simulink model "Distribution_Library"  (Simulink 8.3)
settings: Solver=VariableStepDiscrete  StartTime=0.0  StopTime=100.0  RelTol=1e-3
libraries: simeventslib x4
settings Model: Creator=tsprock3  LastModifiedBy=tsprock3  CovSFcnEnable=on
settings OptimizationCC: ExpressionDepthLimit=2147483647
settings DebuggingCC: FcnCallInpInsideContextMsg=EnableAllAsWarning  FrameProcessingCompatibilityMsg=error  SimStateOlderReleaseMsg=warning
settings GRTTargetCC: CombineOutputUpdateFcns=on  GRTInterface=off

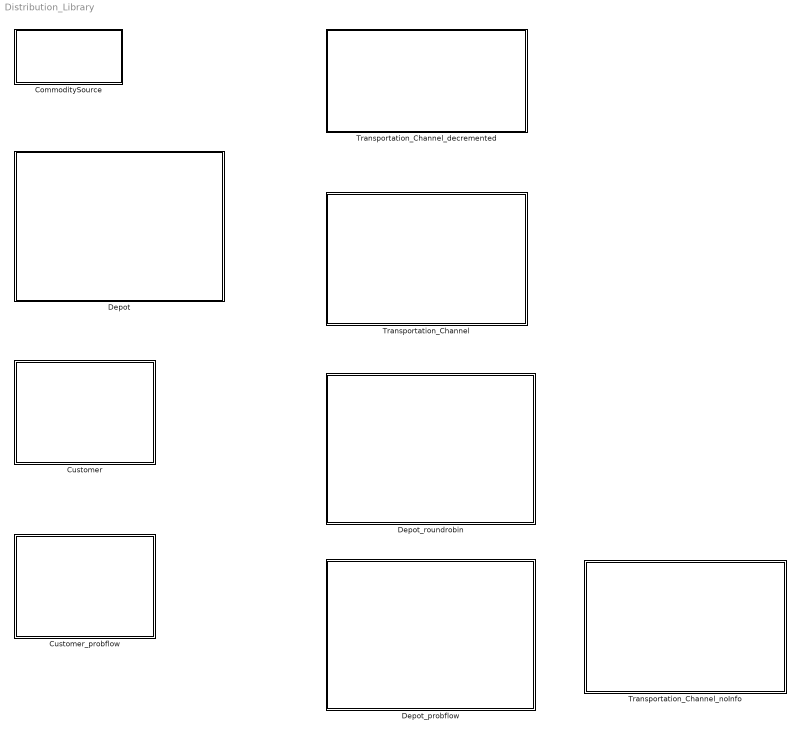
== system Distribution_Library ==
  CommoditySource : Subsystem  mask{Mean=1000/913, AttributeValue=[1 10 9 2]|1|2|1}
      mask prompts: Mean "Frequency"; AttributeValue "Attributes"
      mask TypeOptions Mean: Source/Mean
      mask TypeOptions AttributeValue: setAttribute/AttributeValue
  Customer : Subsystem
  Customer_probflow : Subsystem
  Depot : Subsystem
  Depot_probflow : Subsystem
  Depot_roundrobin : Subsystem
  Transportation_Channel : Subsystem
  Transportation_Channel_decremented : Subsystem
  Transportation_Channel_noInfo : Subsystem

== system Distribution_Library/CommoditySource ==
  Clock : Clock
  Source : TimeBasedEntityGenerator  Distribution=Exponential  InitialSeed=18340  Mean=Mean  GenerateEntityAtSimulationStart=off
  Timed to Event Signal : TimedToEventSignal
  setAttribute : SetAttribute  AttributeName=Route|Origin|Destination|Start  AttributeFrom=Dialog|Dialog|Dialog|Signal port  AttributeValue=[1 10 9 2]|1|2|1  AttributeTreatAsVector=0|1|1|1  EvaluatedAttributeValue={[1 10 9 2];1;2;[]}
      settings: InputPortMap=u3
  OUT_Commodity : PMIOPort  Port=1  Side=Right
  wires:
  Clock/1 -> Timed to Event Signal/1
  Timed to Event Signal/1 -> setAttribute/1
  connections:
  Source/RConn1 -- setAttribute/LConn1
  OUT_Commodity/RConn1 -- setAttribute/RConn1

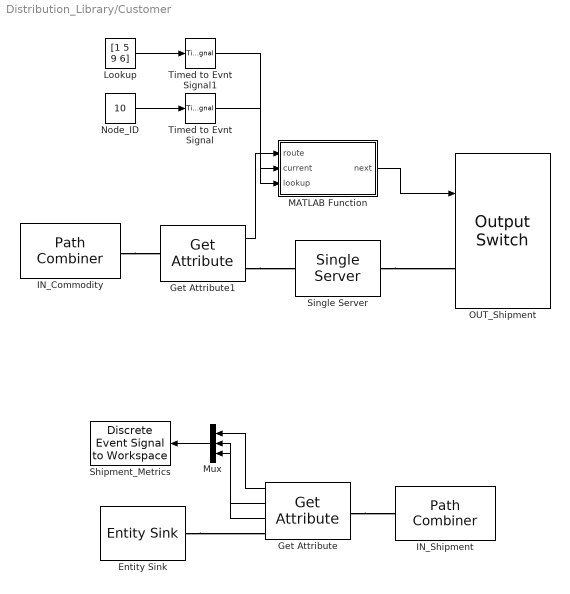
== system Distribution_Library/Customer ==
  Entity Sink : EntitySink
  Get Attribute : GetAttribute  AttributeName=Origin|Destination|Start  AttributeMissing=Error|Error|Error  AttributeDefaultValue=1|1|1  AttributeTreatAsVector=1|1|1  AttributeSendTiming=After entity departure|After entity departure|After entity departure  EvaluatedDefaultAttributeValue={[];[];[]}
      settings: OutputPortMap=o1,o2,o3
  Get Attribute1 : GetAttribute  AttributeName=Route  EvaluatedDefaultAttributeValue={[]}
      settings: OutputPortMap=o1
  IN_Commodity : PathCombiner  NumberInputPorts=4
  IN_Shipment : PathCombiner  NumberInputPorts=1
  Lookup : Constant  Value=[1 5 9 6]
  MATLAB Function : MATLAB Function  TreatAsAtomicUnit=on
  Mux : Mux  Inputs=3
  Node_ID : Constant  Value=10
  OUT_Shipment : OutputSwitch  NumberOutputPorts=1  SwitchingCriterion=From signal port p  AttributeName=Customer
  Shipment_Metrics : simeventslib/SimEvents Sinks/Discrete Event Signal to Workspace  VariableName=Customer_1  SaveFormat=Structure With Time  isMonitorOnly=off  isRecordIC=off
  Single Server : SingleServer  ServiceTime=0
  Timed to Evnt Signal : TimedToEventSignal
  Timed to Evnt Signal1 : TimedToEventSignal
  wires:
  Get Attribute/1 -> Mux/1
  Get Attribute/2 -> Mux/2
  Get Attribute/3 -> Mux/3
  Mux/1 -> Shipment_Metrics/1
  Node_ID/1 -> Timed to Evnt Signal/1
  MATLAB Function/1(next) -> OUT_Shipment/1
  Get Attribute1/1 -> MATLAB Function/1(route)
  Timed to Evnt Signal/1 -> MATLAB Function/2(current)
  Lookup/1 -> Timed to Evnt Signal1/1
  Timed to Evnt Signal1/1 -> MATLAB Function/3(lookup)
  connections:
  Entity Sink/LConn1 -- Get Attribute/RConn1
  Get Attribute/LConn1 -- IN_Shipment/RConn1
  IN_Commodity/RConn1 -- Get Attribute1/LConn1
  Get Attribute1/RConn1 -- Single Server/LConn1
  Single Server/RConn1 -- OUT_Shipment/LConn1

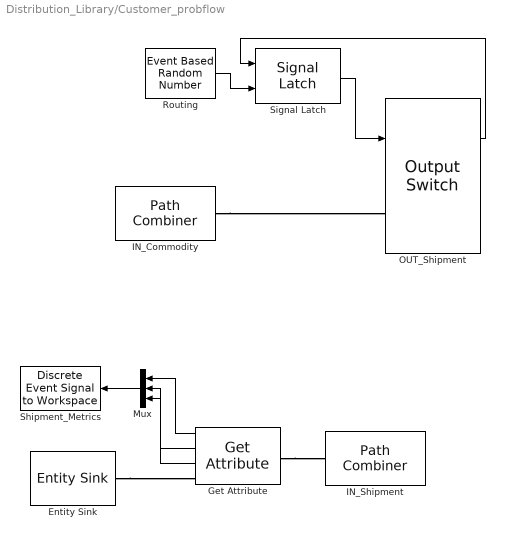
== system Distribution_Library/Customer_probflow ==
  Entity Sink : EntitySink
  Get Attribute : GetAttribute  AttributeName=Origin|Destination|Start  AttributeMissing=Error|Error|Error  AttributeDefaultValue=1|1|1  AttributeTreatAsVector=1|1|1  AttributeSendTiming=After entity departure|After entity departure|After entity departure  EvaluatedDefaultAttributeValue={[];[];[]}
      settings: OutputPortMap=o1,o2,o3
  IN_Commodity : PathCombiner  NumberInputPorts=1
  IN_Shipment : PathCombiner  NumberInputPorts=1
  Mux : Mux  Inputs=3
  OUT_Shipment : OutputSwitch  NumberOutputPorts=1  SwitchingCriterion=From signal port p  AttributeName=Customer  StatNumberDeparted=on
  Routing : EventBasedRandomNumber  Distribution=Arbitrary discrete  valueVecDisc=[1 2]  probVecDisc=[0.1892 0.8108]
  Shipment_Metrics : simeventslib/SimEvents Sinks/Discrete Event Signal to Workspace  VariableName=Customer_1  SaveFormat=Structure With Time  isMonitorOnly=off  isRecordIC=off
  Signal Latch : SignalLatch  InitialMemoryValue=1  ReadMemoryUpon=Write to memory event
      settings: InputPortMap=u0,u2  OutputPortMap=o2
  wires:
  Get Attribute/1 -> Mux/1
  Get Attribute/2 -> Mux/2
  Get Attribute/3 -> Mux/3
  Mux/1 -> Shipment_Metrics/1
  Routing/1 -> Signal Latch/2
  OUT_Shipment/1 -> Signal Latch/1
  Signal Latch/1 -> OUT_Shipment/1
  connections:
  Entity Sink/LConn1 -- Get Attribute/RConn1
  Get Attribute/LConn1 -- IN_Shipment/RConn1
  IN_Commodity/RConn1 -- OUT_Shipment/LConn1

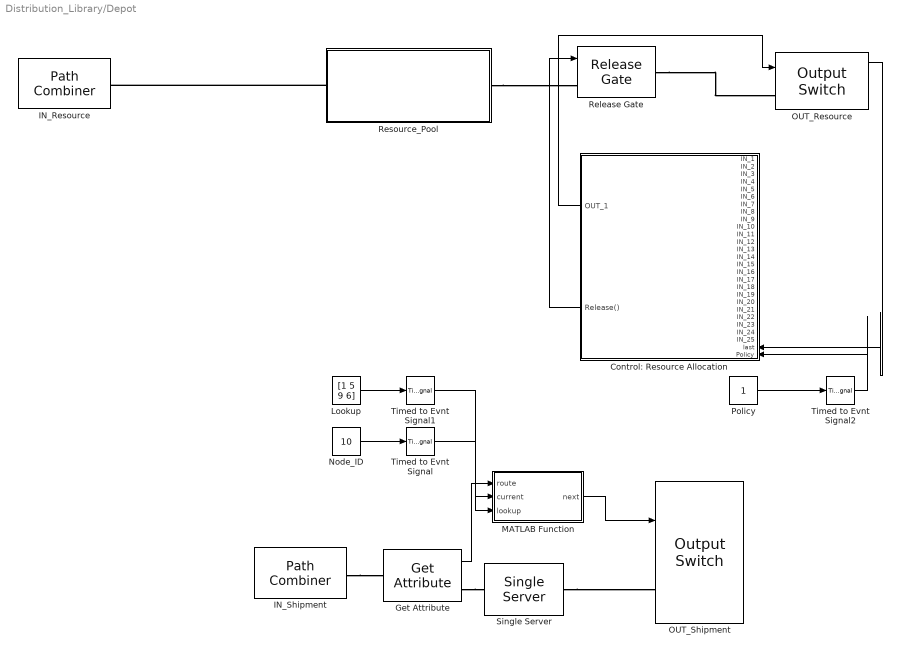
== system Distribution_Library/Depot ==
  Control: Resource Allocation : MATLAB Function  TreatAsAtomicUnit=on
  Get Attribute : GetAttribute  AttributeName=Route  EvaluatedDefaultAttributeValue={[]}
      settings: OutputPortMap=o1
  IN_Resource : PathCombiner  NumberInputPorts=4
  IN_Shipment : PathCombiner  NumberInputPorts=4
  Lookup : Constant  Value=[1 5 9 6]
  MATLAB Function : MATLAB Function  TreatAsAtomicUnit=on
  Node_ID : Constant  Value=10
  OUT_Resource : OutputSwitch  NumberOutputPorts=4  SwitchingCriterion=From signal port p  InitialSeed=57769  StatLastDeparturePort=on
      settings: OutputPortMap=o3
  OUT_Shipment : OutputSwitch  NumberOutputPorts=4  SwitchingCriterion=From signal port p  AttributeName=Customer
  Policy : Constant
  Release Gate : ReleaseGate  OpenGateUpon=Function call from port fcn
  Resource_Pool : Subsystem  mask{Quantity=6}
      mask prompts: Quantity "How many entities in resource pool?"
      mask TypeOptions Quantity:
      | Time-Based
      | Function-Call Generator/NumberOfEventsPerPeriod
  Single Server : SingleServer  ServiceTime=0
  Timed to Evnt Signal : TimedToEventSignal
  Timed to Evnt Signal1 : TimedToEventSignal
  Timed to Evnt Signal2 : TimedToEventSignal
  wires:
  Node_ID/1 -> Timed to Evnt Signal/1
  MATLAB Function/1(next) -> OUT_Shipment/1
  Get Attribute/1 -> MATLAB Function/1(route)
  Timed to Evnt Signal/1 -> MATLAB Function/2(current)
  Lookup/1 -> Timed to Evnt Signal1/1
  Timed to Evnt Signal1/1 -> MATLAB Function/3(lookup)
  Control: Resource Allocation/1(OUT_1) -> OUT_Resource/1
  Control: Resource Allocation/2(Release()) -> Release Gate/1
  OUT_Resource/1 -> Control: Resource Allocation/26(last)
  Policy/1 -> Timed to Evnt Signal2/1
  Timed to Evnt Signal2/1 -> Control: Resource Allocation/27(Policy)
  connections:
  Resource_Pool/RConn1 -- IN_Resource/RConn1
  IN_Shipment/RConn1 -- Get Attribute/LConn1
  Get Attribute/RConn1 -- Single Server/LConn1
  Single Server/RConn1 -- OUT_Shipment/LConn1
  Resource_Pool/LConn1 -- Release Gate/LConn1
  Release Gate/RConn1 -- OUT_Resource/LConn1

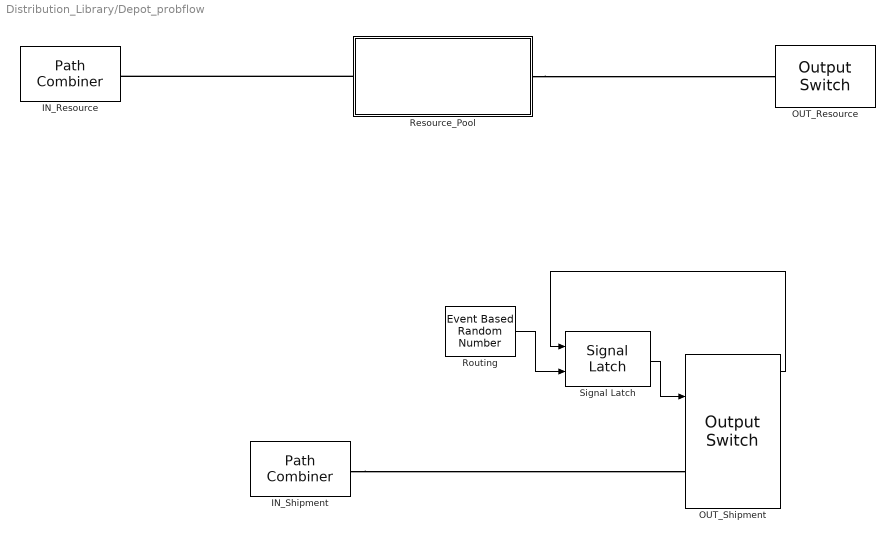
== system Distribution_Library/Depot_probflow ==
  IN_Resource : PathCombiner  NumberInputPorts=4
  IN_Shipment : PathCombiner  NumberInputPorts=4
  OUT_Resource : OutputSwitch  NumberOutputPorts=4  SwitchingCriterion=Round robin  InitialSeed=57769  StatLastDeparturePort=on
      settings: OutputPortMap=o3
  OUT_Shipment : OutputSwitch  NumberOutputPorts=4  SwitchingCriterion=From signal port p  AttributeName=Customer  StatNumberDeparted=on
  Resource_Pool : Subsystem  mask{Quantity=6}
      mask prompts: Quantity "How many entities in resource pool?"
      mask TypeOptions Quantity:
      | Time-Based
      | Function-Call Generator/NumberOfEventsPerPeriod
  Routing : EventBasedRandomNumber  Distribution=Arbitrary discrete  valueVecDisc=[1 2]  probVecDisc=[0.1892 0.8108]
  Signal Latch : SignalLatch  InitialMemoryValue=1  ReadMemoryUpon=Write to memory event
      settings: InputPortMap=u0,u2  OutputPortMap=o2
  wires:
  Signal Latch/1 -> OUT_Shipment/1
  Routing/1 -> Signal Latch/2
  OUT_Shipment/1 -> Signal Latch/1
  connections:
  Resource_Pool/RConn1 -- IN_Resource/RConn1
  IN_Shipment/RConn1 -- OUT_Shipment/LConn1
  Resource_Pool/LConn1 -- OUT_Resource/LConn1

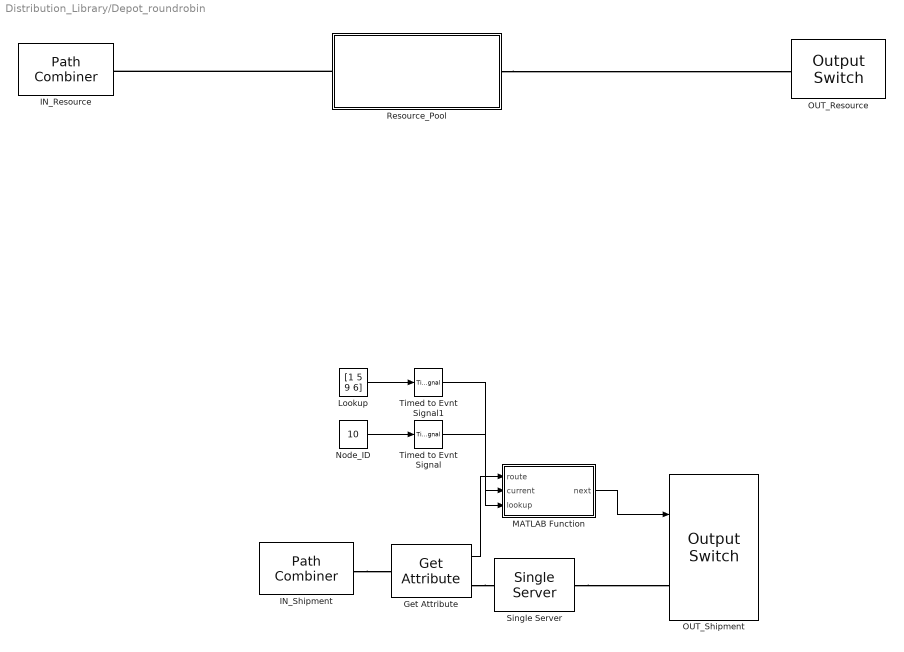
== system Distribution_Library/Depot_roundrobin ==
  Get Attribute : GetAttribute  AttributeName=Route  EvaluatedDefaultAttributeValue={[]}
      settings: OutputPortMap=o1
  IN_Resource : PathCombiner  NumberInputPorts=4
  IN_Shipment : PathCombiner  NumberInputPorts=4
  Lookup : Constant  Value=[1 5 9 6]
  MATLAB Function : MATLAB Function  TreatAsAtomicUnit=on
  Node_ID : Constant  Value=10
  OUT_Resource : OutputSwitch  NumberOutputPorts=4  SwitchingCriterion=Round robin  InitialSeed=57769
  OUT_Shipment : OutputSwitch  NumberOutputPorts=4  SwitchingCriterion=From signal port p  AttributeName=Customer
  Resource_Pool : Subsystem  mask{Quantity=6}
      mask prompts: Quantity "How many entities in resource pool?"
      mask TypeOptions Quantity:
      | Time-Based
      | Function-Call Generator/NumberOfEventsPerPeriod
  Single Server : SingleServer  ServiceTime=0
  Timed to Evnt Signal : TimedToEventSignal
  Timed to Evnt Signal1 : TimedToEventSignal
  wires:
  Node_ID/1 -> Timed to Evnt Signal/1
  MATLAB Function/1(next) -> OUT_Shipment/1
  Get Attribute/1 -> MATLAB Function/1(route)
  Timed to Evnt Signal/1 -> MATLAB Function/2(current)
  Lookup/1 -> Timed to Evnt Signal1/1
  Timed to Evnt Signal1/1 -> MATLAB Function/3(lookup)
  connections:
  Resource_Pool/RConn1 -- IN_Resource/RConn1
  IN_Shipment/RConn1 -- Get Attribute/LConn1
  Get Attribute/RConn1 -- Single Server/LConn1
  Single Server/RConn1 -- OUT_Shipment/LConn1
  Resource_Pool/LConn1 -- OUT_Resource/LConn1

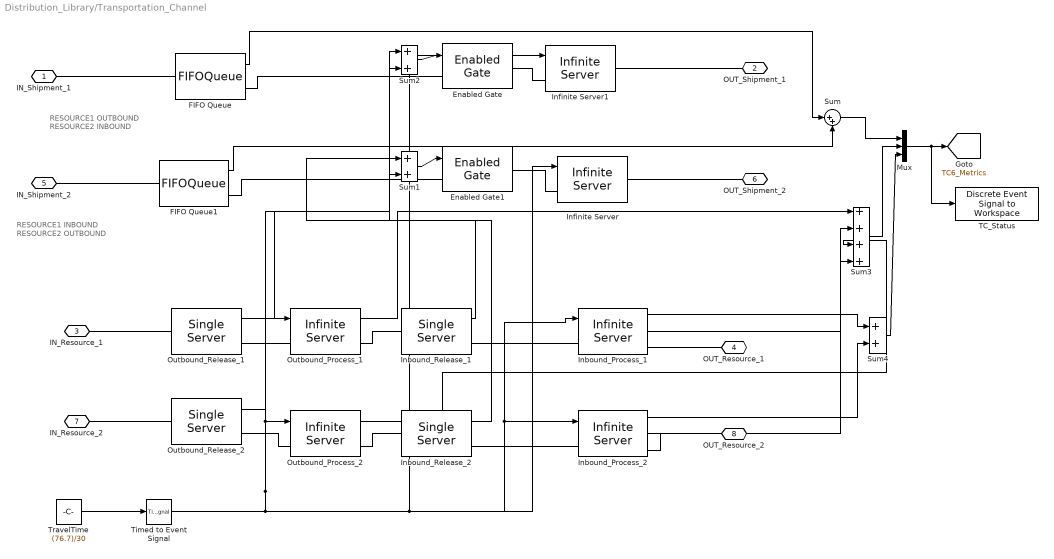
== system Distribution_Library/Transportation_Channel ==
  note: RESOURCE1 INBOUND
      | RESOURCE2 OUTBOUND
  note: RESOURCE1 OUTBOUND
      | RESOURCE2 INBOUND
  Enabled Gate : EnabledGate
  Enabled Gate1 : EnabledGate
  FIFO Queue : FIFOQueue  Capacity=inf  StatNumberInBlock=on
      settings: OutputPortMap=o1
  FIFO Queue1 : FIFOQueue  Capacity=inf  StatNumberInBlock=on
      settings: OutputPortMap=o1
  Inbound_Process_1 : InfiniteServer  ServiceTimeFrom=Signal port t  ServiceTime=(76.7)/30  StatNumberDeparted=on  StatNumberInBlock=on
      settings: OutputPortMap=o0,o1
  Inbound_Process_2 : InfiniteServer  ServiceTimeFrom=Signal port t  ServiceTime=(76.7)/30  StatNumberDeparted=on  StatNumberInBlock=on
      settings: OutputPortMap=o0,o1
  Inbound_Release_1 : SingleServer  ServiceTime=0  StatNumberInBlock=on
      settings: OutputPortMap=o1
  Inbound_Release_2 : SingleServer  ServiceTime=0  StatNumberInBlock=on
      settings: OutputPortMap=o1
  Infinite Server : InfiniteServer  ServiceTimeFrom=Signal port t  ServiceTime=(76.7)/30
  Infinite Server1 : InfiniteServer  ServiceTimeFrom=Signal port t  ServiceTime=(76.7)/30
  Mux : Mux  Inputs=3
  Outbound_Process_1 : InfiniteServer  ServiceTimeFrom=Signal port t  ServiceTime=(76.7)/30  StatNumberInBlock=on
      settings: OutputPortMap=o1
  Outbound_Process_2 : InfiniteServer  ServiceTimeFrom=Signal port t  ServiceTime=(76.7)/30  StatNumberInBlock=on
      settings: OutputPortMap=o1
  Outbound_Release_1 : SingleServer  ServiceTime=0  StatNumberInBlock=on
      settings: OutputPortMap=o1
  Outbound_Release_2 : SingleServer  ServiceTime=0  StatNumberInBlock=on
      settings: OutputPortMap=o1
  Sum{,1..2,4} (4 alike) : Sum  Inputs=|++
  Sum3 : Sum  Inputs=|++++
  TC_Status : simeventslib/SimEvents Sinks/Discrete Event Signal to Workspace  VariableName=TC6_Status  SaveFormat=Structure With Time  isMonitorOnly=off  isRecordIC=off
  Timed to Event Signal : TimedToEventSignal
  TravelTime : Constant  Value=(76.7)/30
  IN_Shipment_1 : PMIOPort  Port=1  Side=Left
  OUT_Shipment_1 : PMIOPort  Port=2  Side=Right
  IN_Resource_1 : PMIOPort  Port=3  Side=Left
  OUT_Resource_1 : PMIOPort  Port=4  Side=Right
  IN_Shipment_2 : PMIOPort  Port=5  Side=Left
  OUT_Shipment_2 : PMIOPort  Port=6  Side=Right
  IN_Resource_2 : PMIOPort  Port=7  Side=Left
  OUT_Resource_2 : PMIOPort  Port=8  Side=Right
  tag scope: TC6_Metrics=global
  wires:
  FIFO Queue1/1 -> Sum/2
  FIFO Queue/1 -> Sum/1
  TravelTime/1 -> Timed to Event Signal/1
  Timed to Event Signal/1 -> Outbound_Process_1/1, Outbound_Process_2/1, Infinite Server1/1, Inbound_Process_1/1, Inbound_Process_2/1, Infinite Server/1
  Sum1/1 -> Enabled Gate1/1
  Outbound_Release_2/1 -> Sum1/2
  Inbound_Release_1/1 -> Sum1/1
  Sum2/1 -> Enabled Gate/1
  Outbound_Release_1/1 -> Sum2/1
  Inbound_Release_2/1 -> Sum2/2
  Mux/1 -> [TC6_Metrics], TC_Status/1
  Sum/1 -> Mux/1
  Sum3/1 -> Mux/2
  Outbound_Process_1/1 -> Sum3/1
  Inbound_Process_1/2 -> Sum3/2
  Outbound_Process_2/1 -> Sum3/3
  Inbound_Process_2/2 -> Sum3/4
  Inbound_Process_1/1 -> Sum4/1
  Inbound_Process_2/1 -> Sum4/2
  Sum4/1 -> Mux/3
  connections:
  FIFO Queue/RConn1 -- Enabled Gate/LConn1
  Enabled Gate1/LConn1 -- FIFO Queue1/RConn1
  IN_Shipment_1/RConn1 -- FIFO Queue/LConn1
  IN_Shipment_2/RConn1 -- FIFO Queue1/LConn1
  IN_Resource_1/RConn1 -- Outbound_Release_1/LConn1
  OUT_Shipment_2/RConn1 -- Infinite Server/RConn1
  Infinite Server/LConn1 -- Enabled Gate1/RConn1
  Enabled Gate/RConn1 -- Infinite Server1/LConn1
  Infinite Server1/RConn1 -- OUT_Shipment_1/RConn1
  IN_Resource_2/RConn1 -- Outbound_Release_2/LConn1
  Outbound_Release_2/RConn1 -- Outbound_Process_2/LConn1
  Outbound_Process_2/RConn1 -- Inbound_Release_2/LConn1
  Inbound_Release_2/RConn1 -- Inbound_Process_2/LConn1
  Inbound_Process_2/RConn1 -- OUT_Resource_2/RConn1
  Outbound_Release_1/RConn1 -- Outbound_Process_1/LConn1
  Inbound_Release_1/RConn1 -- Inbound_Process_1/LConn1
  Outbound_Process_1/RConn1 -- Inbound_Release_1/LConn1
  Inbound_Process_1/RConn1 -- OUT_Resource_1/RConn1

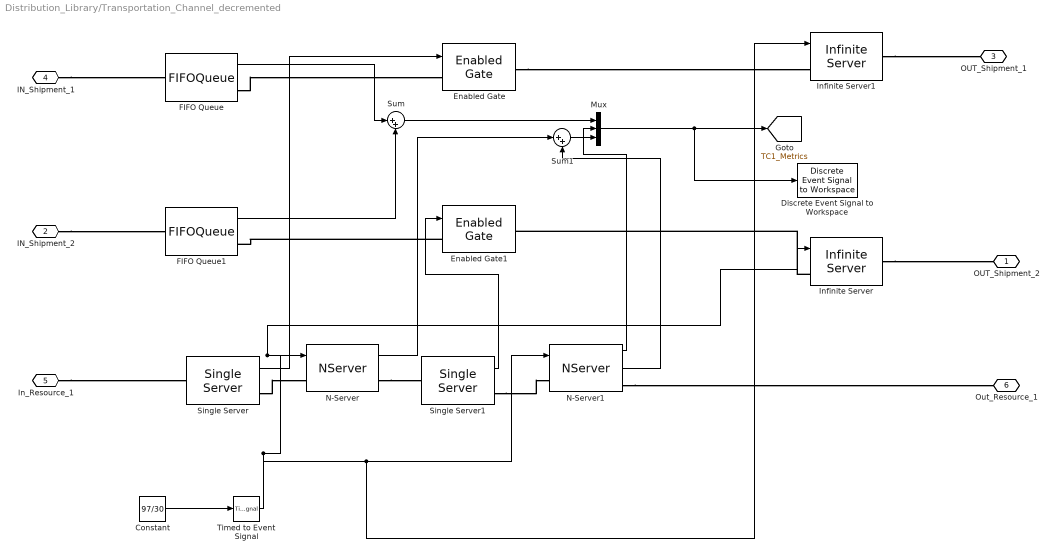
== system Distribution_Library/Transportation_Channel_decremented ==
  Constant : Constant  Value=97/30
  Discrete Event Signal to Workspace : simeventslib/SimEvents Sinks/Discrete Event Signal to Workspace  VariableName=TC1_Status  SaveFormat=Structure With Time  isMonitorOnly=off  isRecordIC=off
  Enabled Gate : EnabledGate
  Enabled Gate1 : EnabledGate
  FIFO Queue : FIFOQueue  Capacity=inf  StatNumberInBlock=on
      settings: OutputPortMap=o1
  FIFO Queue1 : FIFOQueue  Capacity=inf  StatNumberInBlock=on
      settings: OutputPortMap=o1
  Infinite Server : InfiniteServer  ServiceTimeFrom=Signal port t
  Infinite Server1 : InfiniteServer  ServiceTimeFrom=Signal port t
  Mux : Mux  Inputs=3
  N-Server : NServer  NumberOfServers=inf  ServiceTimeFrom=Signal port t  StatNumberInBlock=on
      settings: OutputPortMap=o1
  N-Server1 : NServer  NumberOfServers=inf  ServiceTimeFrom=Signal port t  StatNumberDeparted=on  StatNumberInBlock=on
      settings: OutputPortMap=o0,o1
  Single Server : SingleServer  ServiceTime=0  StatNumberInBlock=on
      settings: OutputPortMap=o1
  Single Server1 : SingleServer  ServiceTime=0  StatNumberInBlock=on
      settings: OutputPortMap=o1
  Sum : Sum  Inputs=|++
  Sum1 : Sum  Inputs=|++
  Timed to Event Signal : TimedToEventSignal
  OUT_Shipment_2 : PMIOPort  Port=1  Side=Right
  IN_Shipment_2 : PMIOPort  Port=2  Side=Left
  OUT_Shipment_1 : PMIOPort  Port=3  Side=Left
  IN_Shipment_1 : PMIOPort  Port=4  Side=Right
  In_Resource_1 : PMIOPort  Port=5  Side=Right
  Out_Resource_1 : PMIOPort  Port=6  Side=Right
  tag scope: TC1_Metrics=global
  wires:
  FIFO Queue1/1 -> Sum/2
  FIFO Queue/1 -> Sum/1
  Sum/1 -> Mux/1
  Constant/1 -> Timed to Event Signal/1
  Timed to Event Signal/1 -> Infinite Server/1, N-Server/1, Infinite Server1/1, N-Server1/1
  N-Server/1 -> Sum1/1
  N-Server1/2 -> Sum1/2
  Sum1/1 -> Mux/2
  Mux/1 -> [TC1_Metrics], Discrete Event Signal to Workspace/1
  N-Server1/1 -> Mux/3
  Single Server/1 -> Enabled Gate/1
  Single Server1/1 -> Enabled Gate1/1
  connections:
  FIFO Queue/RConn1 -- Enabled Gate/LConn1
  Enabled Gate1/LConn1 -- FIFO Queue1/RConn1
  Infinite Server/LConn1 -- Enabled Gate1/RConn1
  Enabled Gate/RConn1 -- Infinite Server1/LConn1
  Single Server/RConn1 -- N-Server/LConn1
  N-Server/RConn1 -- Single Server1/LConn1
  Single Server1/RConn1 -- N-Server1/LConn1
  In_Resource_1/RConn1 -- Single Server/LConn1
  N-Server1/RConn1 -- Out_Resource_1/RConn1
  IN_Shipment_1/RConn1 -- FIFO Queue/LConn1
  IN_Shipment_2/RConn1 -- FIFO Queue1/LConn1
  Infinite Server1/RConn1 -- OUT_Shipment_1/RConn1
  Infinite Server/RConn1 -- OUT_Shipment_2/RConn1

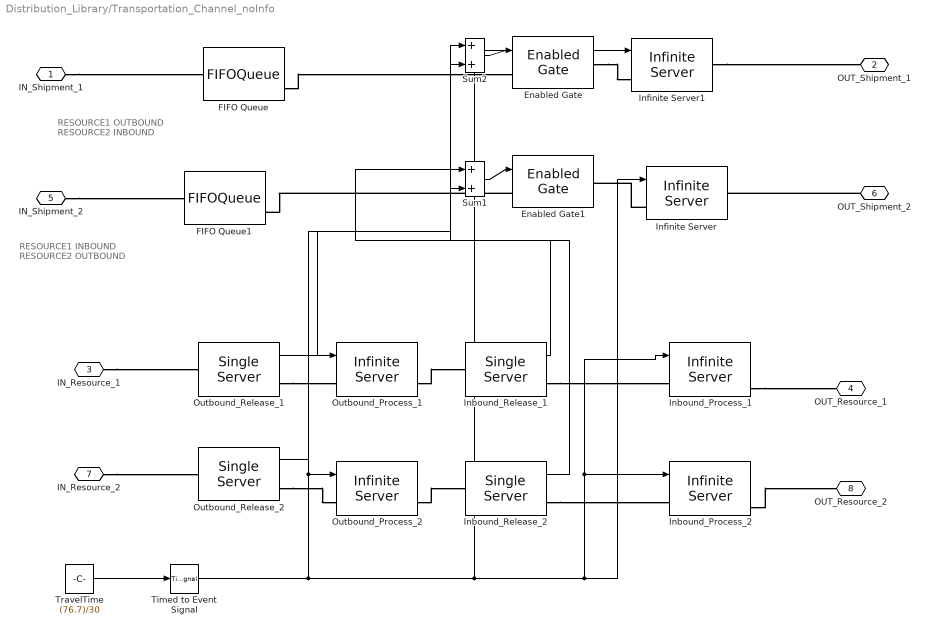
== system Distribution_Library/Transportation_Channel_noInfo ==
  note: RESOURCE1 INBOUND
      | RESOURCE2 OUTBOUND
  note: RESOURCE1 OUTBOUND
      | RESOURCE2 INBOUND
  Enabled Gate : EnabledGate
  Enabled Gate1 : EnabledGate
  FIFO Queue : FIFOQueue  Capacity=inf  StatNumberInBlock=on
      settings: OutputPortMap=o1
  FIFO Queue1 : FIFOQueue  Capacity=inf  StatNumberInBlock=on
      settings: OutputPortMap=o1
  Inbound_Process_1 : InfiniteServer  ServiceTimeFrom=Signal port t  ServiceTime=(76.7)/30  StatNumberDeparted=on  StatNumberInBlock=on
      settings: OutputPortMap=o0,o1
  Inbound_Process_2 : InfiniteServer  ServiceTimeFrom=Signal port t  ServiceTime=(76.7)/30  StatNumberDeparted=on  StatNumberInBlock=on
      settings: OutputPortMap=o0,o1
  Inbound_Release_1 : SingleServer  ServiceTime=0  StatNumberInBlock=on
      settings: OutputPortMap=o1
  Inbound_Release_2 : SingleServer  ServiceTime=0  StatNumberInBlock=on
      settings: OutputPortMap=o1
  Infinite Server : InfiniteServer  ServiceTimeFrom=Signal port t  ServiceTime=(76.7)/30
  Infinite Server1 : InfiniteServer  ServiceTimeFrom=Signal port t  ServiceTime=(76.7)/30
  Outbound_Process_1 : InfiniteServer  ServiceTimeFrom=Signal port t  ServiceTime=(76.7)/30  StatNumberInBlock=on
      settings: OutputPortMap=o1
  Outbound_Process_2 : InfiniteServer  ServiceTimeFrom=Signal port t  ServiceTime=(76.7)/30  StatNumberInBlock=on
      settings: OutputPortMap=o1
  Outbound_Release_1 : SingleServer  ServiceTime=0  StatNumberInBlock=on
      settings: OutputPortMap=o1
  Outbound_Release_2 : SingleServer  ServiceTime=0  StatNumberInBlock=on
      settings: OutputPortMap=o1
  Sum1 : Sum  Inputs=|++
  Sum2 : Sum  Inputs=|++
  Timed to Event Signal : TimedToEventSignal
  TravelTime : Constant  Value=(76.7)/30
  IN_Shipment_1 : PMIOPort  Port=1  Side=Left
  OUT_Shipment_1 : PMIOPort  Port=2  Side=Right
  IN_Resource_1 : PMIOPort  Port=3  Side=Left
  OUT_Resource_1 : PMIOPort  Port=4  Side=Right
  IN_Shipment_2 : PMIOPort  Port=5  Side=Left
  OUT_Shipment_2 : PMIOPort  Port=6  Side=Right
  IN_Resource_2 : PMIOPort  Port=7  Side=Left
  OUT_Resource_2 : PMIOPort  Port=8  Side=Right
  wires:
  TravelTime/1 -> Timed to Event Signal/1
  Timed to Event Signal/1 -> Infinite Server/1, Inbound_Process_1/1, Inbound_Process_2/1, Infinite Server1/1, Outbound_Process_1/1, Outbound_Process_2/1
  Sum1/1 -> Enabled Gate1/1
  Outbound_Release_2/1 -> Sum1/2
  Inbound_Release_1/1 -> Sum1/1
  Sum2/1 -> Enabled Gate/1
  Outbound_Release_1/1 -> Sum2/1
  Inbound_Release_2/1 -> Sum2/2
  connections:
  FIFO Queue/RConn1 -- Enabled Gate/LConn1
  Enabled Gate1/LConn1 -- FIFO Queue1/RConn1
  IN_Shipment_1/RConn1 -- FIFO Queue/LConn1
  IN_Shipment_2/RConn1 -- FIFO Queue1/LConn1
  IN_Resource_1/RConn1 -- Outbound_Release_1/LConn1
  OUT_Shipment_2/RConn1 -- Infinite Server/RConn1
  Infinite Server/LConn1 -- Enabled Gate1/RConn1
  Enabled Gate/RConn1 -- Infinite Server1/LConn1
  Infinite Server1/RConn1 -- OUT_Shipment_1/RConn1
  IN_Resource_2/RConn1 -- Outbound_Release_2/LConn1
  Outbound_Release_2/RConn1 -- Outbound_Process_2/LConn1
  Outbound_Process_2/RConn1 -- Inbound_Release_2/LConn1
  Inbound_Release_2/RConn1 -- Inbound_Process_2/LConn1
  Inbound_Process_2/RConn1 -- OUT_Resource_2/RConn1
  Outbound_Release_1/RConn1 -- Outbound_Process_1/LConn1
  Inbound_Release_1/RConn1 -- Inbound_Process_1/LConn1
  Outbound_Process_1/RConn1 -- Inbound_Release_1/LConn1
  Inbound_Process_1/RConn1 -- OUT_Resource_1/RConn1

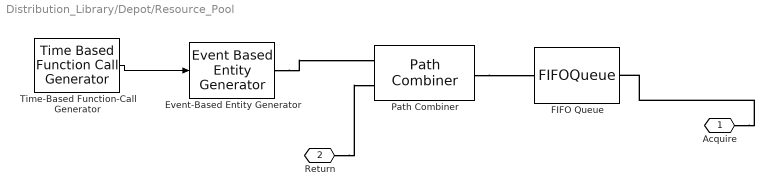
== system Distribution_Library/Depot/Resource_Pool ==
  Event-Based Entity Generator : EventBasedEntityGenerator  GenerateEntitiesUpon=Function call from port fcn
  FIFO Queue : FIFOQueue  Capacity=8
  Path Combiner : PathCombiner  NumberInputPorts=2
  Time-Based Function-Call Generator : TimeBasedFunctionCallGenerator  EventGenerationMode=Only at simulation start  NumberOfEventsPerPeriod=Quantity
  Acquire : PMIOPort  Port=1  Side=Left
  Return : PMIOPort  Port=2  Side=Right
  wires:
  Time-Based Function-Call Generator/1 -> Event-Based Entity Generator/1
  connections:
  Event-Based Entity Generator/RConn1 -- Path Combiner/LConn1
  Path Combiner/RConn1 -- FIFO Queue/LConn1
  Return/RConn1 -- Path Combiner/LConn2
  Acquire/RConn1 -- FIFO Queue/RConn1

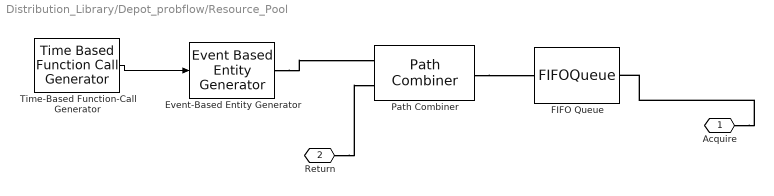
== system Distribution_Library/Depot_probflow/Resource_Pool ==
  Event-Based Entity Generator : EventBasedEntityGenerator  GenerateEntitiesUpon=Function call from port fcn
  FIFO Queue : FIFOQueue  Capacity=8
  Path Combiner : PathCombiner  NumberInputPorts=2
  Time-Based Function-Call Generator : TimeBasedFunctionCallGenerator  EventGenerationMode=Only at simulation start  NumberOfEventsPerPeriod=Quantity
  Acquire : PMIOPort  Port=1  Side=Left
  Return : PMIOPort  Port=2  Side=Right
  wires:
  Time-Based Function-Call Generator/1 -> Event-Based Entity Generator/1
  connections:
  Event-Based Entity Generator/RConn1 -- Path Combiner/LConn1
  Path Combiner/RConn1 -- FIFO Queue/LConn1
  Return/RConn1 -- Path Combiner/LConn2
  Acquire/RConn1 -- FIFO Queue/RConn1

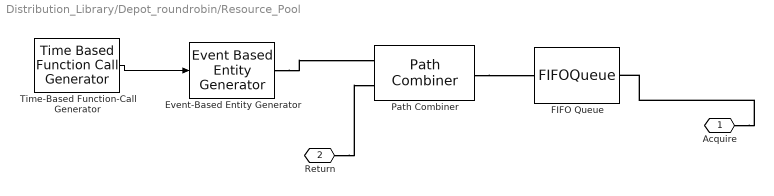
== system Distribution_Library/Depot_roundrobin/Resource_Pool ==
  Event-Based Entity Generator : EventBasedEntityGenerator  GenerateEntitiesUpon=Function call from port fcn
  FIFO Queue : FIFOQueue  Capacity=8
  Path Combiner : PathCombiner  NumberInputPorts=2
  Time-Based Function-Call Generator : TimeBasedFunctionCallGenerator  EventGenerationMode=Only at simulation start  NumberOfEventsPerPeriod=Quantity
  Acquire : PMIOPort  Port=1  Side=Left
  Return : PMIOPort  Port=2  Side=Right
  wires:
  Time-Based Function-Call Generator/1 -> Event-Based Entity Generator/1
  connections:
  Event-Based Entity Generator/RConn1 -- Path Combiner/LConn1
  Path Combiner/RConn1 -- FIFO Queue/LConn1
  Return/RConn1 -- Path Combiner/LConn2
  Acquire/RConn1 -- FIFO Queue/RConn1

== matlab function Customer/MATLAB Function ==
  data: route input double; next output double; current input double; lookup input double
function next = routing(route, current, lookup)
%#codegen
next = 1;
for i = 1:length(route)
   if route(i) == current
       next = route(i+1);
   end
   
   for j = 1:length(lookup)
       if lookup(j) == next
           next = j;
       end
   end
end

== matlab function Depot/MATLAB Function ==
  data: route input double; next output double; current input double; lookup input double
function next = routing(route, current, lookup)
%#codegen
next = 1;
for i = 1:length(route)
   if route(i) == current
       next = route(i+1);
   end
   
   for j = 1:length(lookup)
       if lookup(j) == next
           next = j;
       end
   end
end

== matlab function Depot/Control: Resource Allocation ==
  data: IN_1 input double; OUT_1 output double; IN_2 input double; IN_3 input double; IN_4 input double; IN_5 input double; IN_6 input double; IN_7 input double; IN_8 input double; IN_9 input double; IN_10 input double; IN_11 input double; IN_12 input double; IN_13 input double; IN_14 input double; IN_15 input double; IN_16 input double; IN_17 input double; IN_18 input double; IN_19 input double; IN_20 input double; IN_21 input double; IN_22 input double; IN_23 input double; IN_24 input double; IN_25 input double; last input double; Policy input double
  events: Release output FUNCTION_CALL_EVENT
function OUT_1 = resource_alloc(IN_1, IN_2, IN_3, IN_4, IN_5, IN_6, IN_7, IN_8, IN_9, IN_10, IN_11, IN_12, IN_13, IN_14, IN_15, IN_16, IN_17, IN_18, IN_19, IN_20, IN_21, IN_22, IN_23, IN_24, IN_25, last, Policy)
%#codegen

OUT_1 = 1;

if last ==0
    last =1;
end

%Policy 1 := 'Longest Queue';
%Policy 2 := 'Minimum Queue';
%Policy default := 'Round Robin';
Status = zeros(25,3);

if length(IN_25)>1
    Status(25,:) = [IN_25'];
else
    Status = zeros(24,3);
end
if length(IN_24)>1
    Status(24,:) = [IN_24'];
else
    Status = zeros(23,3);
end
if length(IN_23)>1
    Status(23,:) = [IN_23'];
else
    Status = zeros(22,3);
end
if length(IN_22)>1
    Status(22,:) = [IN_22'];
else
    Status = zeros(21,3);
end
if length(IN_21)>1
    Status(21,:) = [IN_21'];
else
    Status = zeros(20,3);
end
if length(IN_20)>1
    Status(20,:) = [IN_20'];
else
    Status = zeros(19,3);
end
if length(IN_19)>1
    Status(19,:) = [IN_19'];
else
    Status = zeros(18,3);
end
if length(IN_18)>1
    Status(18,:) = [IN_18'];
else
    Status = zeros(17,3);
end
if length(IN_17)>1
    Status(17,:) = [IN_17'];
else
    Status = zeros(16,3);
end
if length(IN_16)>1
    Status(16,:) = [IN_16'];
else
    Status = zeros(15,3);
end
if length(IN_15)>1
    Status(15,:) = [IN_15'];
else
    Status = zeros(14,3);
end
if length(IN_14)>1
    Status(14,:) = [IN_14'];
else
    Status = zeros(13,3);
end
if length(IN_13)>1
    Status(13,:) = [IN_13'];
else
    Status = zeros(12,3);
end
if length(IN_12)>1
    Status(12,:) = [IN_12'];
else
    Status = zeros(11,3);
end
if length(IN_11)>1
    Status(11,:) = [IN_11'];
else
    Status = zeros(10,3);
end
if length(IN_10)>1
    Status(10,:) = [IN_10'];
else
    Status = zeros(9,3);
end
if length(IN_9)>1
    Status(9,:) = [IN_9'];
else
    Status = zeros(8,3);
end
if length(IN_8)>1
    Status(8,:) = [IN_8'];
else
    Status = zeros(7,3);
end
if length(IN_7)>1
    Status(7,:) = [IN_7'];
else
    Status = zeros(6,3);
end
if length(IN_6)>1
    Status(6,:) = [IN_6'];
else
    Status = zeros(5,3);
end

if length(IN_5)>1
    Status(5,:) = [IN_5'];
else
    Status = zeros(4,3);
end
if length(IN_4)>1
    Status(4,:) = [IN_4'];
else
    Status = zeros(3,3);
end
if length(IN_3)>1
    Status(3,:) = [IN_3'];
else
    Status = zeros(2,3);
end
if length(IN_2)>1
    Status(2,:) = [IN_2'];
else
    Status = zeros(1,3);
end

Status(1,:) = [IN_1'];

        


if eq(Policy, 1) ==1
    Status(last, :) = [NaN, NaN, NaN];
    y = min(Status(:,2));
    x = max(Status(Status(:,2)==y));

    for i = 1:length(Status(:,1))
       if Status(i,1)== x && Status(i,2) == y
           Release;
           OUT_1 = i;
           last = i;
           break;
       end
    end
    
elseif eq(Policy, 2) ==1
    Status(last, :) = [NaN, NaN, NaN];
    y = min(Status(:,2));
    x = max(Status(Status(:,2)==y));

    for i = 1:length(Status(:,1))
       if Status(i,1)== x && Status(i,2) == y && Status(i,1)>10 && Status(i,2)<2
           Release;
           OUT_1 = i;
           last =i;
           break;
       end
    end
else %Round-Robin
    PortCount = length(Status);
    
    if last == PortCount
        OUT_1 = 1;
        last = last+1;
    else
        OUT_1 = last +1;
        last = last+1;
    end
    Release;
end

== matlab function Depot_roundrobin/MATLAB Function ==
  data: route input double; next output double; current input double; lookup input double
function next = routing(route, current, lookup)
%#codegen
next = 1;
for i = 1:length(route)
   if route(i) == current
       next = route(i+1);
   end
   
   for j = 1:length(lookup)
       if lookup(j) == next
           next = j;
       end
   end
end
